simulink model "threephase_rl_full"  (R2013b)
settings: Solver=ode45  StartTime=0.0  StopTime=0.04  RelTol=1e-3
undefined symbols (not defined in the file): alpha
libraries: powerlib x27
settings Model: Creator=SAI KUMAR  LastModifiedBy=SAI KUMAR

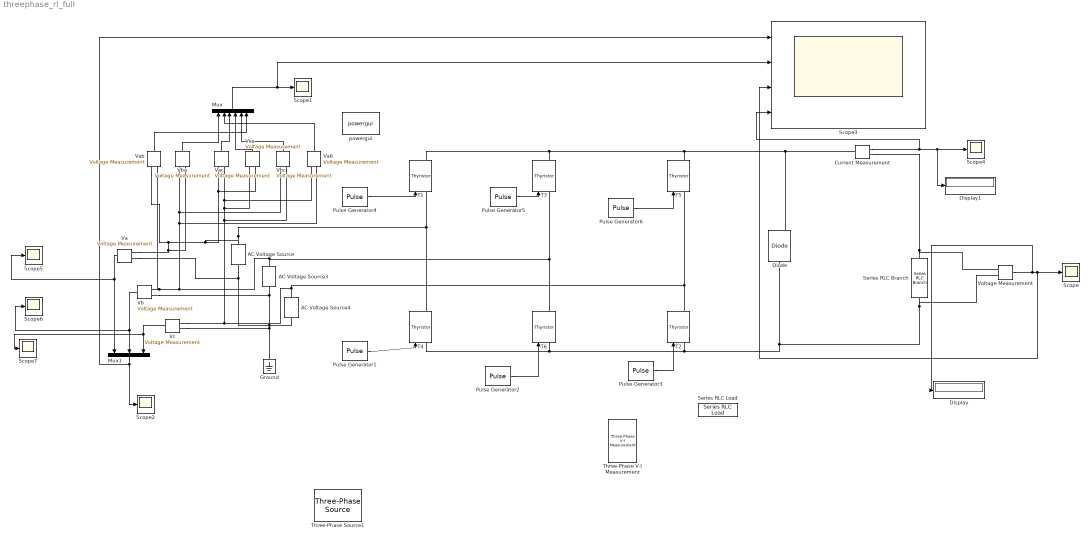
== system threephase_rl_full ==
  AC Voltage Source : powerlib/Electrical Sources/AC Voltage Source  Amplitude=220*sqrt(2)  Phase=0  Frequency=50  SampleTime=0  Measurements=None
  AC Voltage Source3 : powerlib/Electrical Sources/AC Voltage Source  Amplitude=220*sqrt(2)  Phase=-120  Frequency=50  SampleTime=0  Measurements=None
  AC Voltage Source4 : powerlib/Electrical Sources/AC Voltage Source  Amplitude=220*sqrt(2)  Phase=120  Frequency=50  SampleTime=0  Measurements=None
  Current Measurement : powerlib/Measurements/Current Measurement  PhasorSimulation=off  OutputType=Complex  PSBequivalent=0
  Diode : powerlib/Power Electronics/Diode  Ron=0.001  Lon=0  Vf=0.8  IC=0  UseSnubber=off  Rs=500  Cs=250e-9  Measurements=on
  Display : Display
  Display1 : Display
  Ground : powerlib/Elements/Ground  LConnTagsString=a
  Mux : Mux  Inputs=6
  Mux1 : Mux  Inputs=3
  Pulse Generator1 : DiscretePulseGenerator  PulseType=Time based  Amplitude=2  Period=.02  PulseWidth=100/3  PhaseDelay=.011666667+(.02/360)*alpha
  Pulse Generator2 : DiscretePulseGenerator  PulseType=Time based  Amplitude=2  Period=.02  PulseWidth=100/3  PhaseDelay=0.018333+(.02/360)*alpha
  Pulse Generator3 : DiscretePulseGenerator  PulseType=Time based  Amplitude=2  Period=.02  PulseWidth=100/3  PhaseDelay=.005+(.02/360)*alpha
  Pulse Generator4 : DiscretePulseGenerator  PulseType=Time based  Amplitude=2  Period=.02  PulseWidth=100/3  PhaseDelay=.00166666+(.02/360)*alpha
  Pulse Generator5 : DiscretePulseGenerator  PulseType=Time based  Amplitude=2  Period=.02  PulseWidth=100/3  PhaseDelay=.0083333+(.02/360)*alpha
  Pulse Generator6 : DiscretePulseGenerator  PulseType=Time based  Amplitude=2  Period=.02  PulseWidth=100/3  PhaseDelay=.015+(.02/360)*alpha
  Scope{,1..2,4..7} (7 alike) : Scope
      Scope settings: TimeRange=1
      Scope2 settings: SaveName=ScopeData2
      Scope4 settings: SaveName=ScopeData4
      Scope5 settings: SaveName=ScopeData5
      Scope6 settings: SaveName=ScopeData6
      Scope7 settings: SaveName=ScopeData7
  Scope3 : Scope  NumInputPorts=4
      settings: ShowLegends=on  YMin=-5~-5~-5~-5  YMax=5~5~5~5  SaveName=ScopeData3
  Series RLC Branch : powerlib/Elements/Series RLC Branch  LConnTagsString=__new0  RConnTagsString=__new0  BranchType=RL  Resistance=15  Inductance=10e-3  SetiL0=off  InitialCurrent=0  Capacitance=1e-6  Setx0=off  InitialVoltage=0  Measurements=None
  Series RLC Load : powerlib/Elements/Series RLC Load  LConnTagsString=a  RConnTagsString=__new0  NominalVoltage=1000  NominalFrequency=60  ActivePower=10e3  InductivePower=100  CapacitivePower=100  Setx0=off  InitialVoltage=0  SetiL0=off  InitialCurrent=0  Measurements=None
  T{1..6} (6 alike) : powerlib/Power Electronics/Thyristor  Ron=0.001  Lon=0  Vf=0.8  IC=0  Rs=500  Cs=250e-9  Measurements=on
  Three-Phase V-I Measurement : powerlib/Measurements/Three-Phase V-I Measurement  VoltageMeasurement=phase-to-ground  SetLabelV=off  LabelV=Vabc  Vpu=off  VpuLL=off  CurrentMeasurement=yes  SetLabelI=off  LabelI=Iabc  Ipu=off  Pbase=100e6  Vbase=500e3  OutputType=Complex  PhasorSimulation=off  PSBequivalent=0
  Three-Phase Source1 : powerlib/Electrical Sources/Three-Phase Source  Voltage=25e3  PhaseAngle=0  Frequency=60  InternalConnection=Yg  SpecifyImpedance=on  Resistance=0.8929  Inductance=16.58e-3  ShortCircuitLevel=100e6  BaseVoltage=25e3  XRratio=0  BusType=swing  Pref=0  Qref=0  Qmin=-inf  Qmax=inf
  Va : powerlib/Measurements/Voltage Measurement  PhasorSimulation=off  OutputType=Complex  PSBequivalent=0
  Va6 : powerlib/Measurements/Voltage Measurement  PhasorSimulation=off  OutputType=Complex  PSBequivalent=0
  Vab : powerlib/Measurements/Voltage Measurement  PhasorSimulation=off  OutputType=Complex  PSBequivalent=0
  Vac : powerlib/Measurements/Voltage Measurement  PhasorSimulation=off  OutputType=Complex  PSBequivalent=0
  Vb : powerlib/Measurements/Voltage Measurement  PhasorSimulation=off  OutputType=Complex  PSBequivalent=0
  Vba : powerlib/Measurements/Voltage Measurement  PhasorSimulation=off  OutputType=Complex  PSBequivalent=0
  Vbc : powerlib/Measurements/Voltage Measurement  PhasorSimulation=off  OutputType=Complex  PSBequivalent=0
  Vc : powerlib/Measurements/Voltage Measurement  PhasorSimulation=off  OutputType=Complex  PSBequivalent=0
  Vca : powerlib/Measurements/Voltage Measurement  PhasorSimulation=off  OutputType=Complex  PSBequivalent=0
  Voltage Measurement : powerlib/Measurements/Voltage Measurement  PhasorSimulation=off  OutputType=Complex  PSBequivalent=0
  powergui : powerlib/powergui  Priority=1  SimulationMode=Continuous  SolverType=Tustin  SampleTime=50e-6  frequency=60  SPID=off  DisableSnubberDevices=off  DisableRonSwitches=off  DisableVfSwitches=off  SwTol=0  Interpol=off  DisplayEquations=off  frequencyindice=50  Pbase=100e6  ErrMax=1e-4  Iterations=50  UnitsV=kV  UnitsW=MW  FunctionMessages=off  echomessages=off  HookPort=off  EnableUseOfTLC=off  x0status=blocks  RestoreLinks=warning  ResistiveCurrentMeasurement=off  Frange=[0:2:500]  Ylog=off  Xlog=on  ShowGrid=off  save=off  variable=ZData  ZoomFFT=off  StartTime=0.0  cycles=1  DisplayStyle=1  fundamental=60  FreqAxis=off  MaxFrequency=1000  frequencyindicesteady=1  RmsSteady=1  display=off  Ts=0  methode=off
  wires:
  Pulse Generator1/1 -> T4/1
  Pulse Generator2/1 -> T6/1
  Pulse Generator3/1 -> T2/1
  Pulse Generator4/1 -> T1/1
  Pulse Generator5/1 -> T3/1
  Pulse Generator6/1 -> T5/1
  Voltage Measurement/1 -> Display/1, Scope3/3, Scope/1
  Vab/1 -> Mux/6
  Vba/1 -> Mux/1
  Vac/1 -> Mux/3
  Vca/1 -> Mux/4
  Vbc/1 -> Mux/5
  Va6/1 -> Mux/2
  Mux/1 -> Scope3/2, Scope1/1
  Va/1 -> Scope5/1, Mux1/1
  Vb/1 -> Scope6/1, Mux1/2
  Vc/1 -> Mux1/3, Scope7/1
  Mux1/1 -> Scope2/1, Scope3/1
  Current Measurement/1 -> Scope3/4, Display1/1, Scope4/1
  connections:
  T1/LConn1 -- T4/RConn1 -- Vca/LConn2 -- Vac/LConn1 -- Vba/LConn2 -- Va/LConn1 -- Vab/LConn1 -- AC Voltage Source/RConn1
  T3/LConn1 -- T6/RConn1 -- Va6/LConn2 -- Vbc/LConn1 -- Vba/LConn1 -- Vab/LConn2 -- Vb/LConn1 -- AC Voltage Source3/RConn1
  T5/LConn1 -- T2/RConn1 -- Vbc/LConn2 -- Va6/LConn1 -- Vac/LConn2 -- Vca/LConn1 -- Vc/LConn1 -- AC Voltage Source4/RConn1
  T6/LConn1 -- T4/LConn1 -- Series RLC Branch/RConn1 -- Voltage Measurement/LConn2 -- Diode/LConn1 -- T2/LConn1
  T5/RConn1 -- Current Measurement/LConn1 -- Diode/RConn1 -- T1/RConn1 -- T3/RConn1
  Voltage Measurement/LConn1 -- Current Measurement/RConn1 -- Series RLC Branch/LConn1
  AC Voltage Source4/LConn1 -- Ground/LConn1 -- Vc/LConn2 -- AC Voltage Source3/LConn1 -- Vb/LConn2 -- AC Voltage Source/LConn1 -- Va/LConn2
